simulink model "Sim_Control_Dezvoltare"  (R2022b)
settings: Solver=VariableStepAuto  StartTime=0.0  StopTime=400  RelTol=1e-3
values from neighbouring files (symbols this model uses):
  g = 9.80665    [Date_initializare_SIM.m]
  h = 0.30    (= 0.3)    [Date_initializare_SIM.m]
undefined symbols (not defined in the file or in its folder): X, Y, Z
libraries: sm_lib x175, nesl_utility x70, slpidlib x2
(part 1 of 5)
settings Model: PacingRate=1.100000  Creator=MUN  LastModifiedBy=MUN

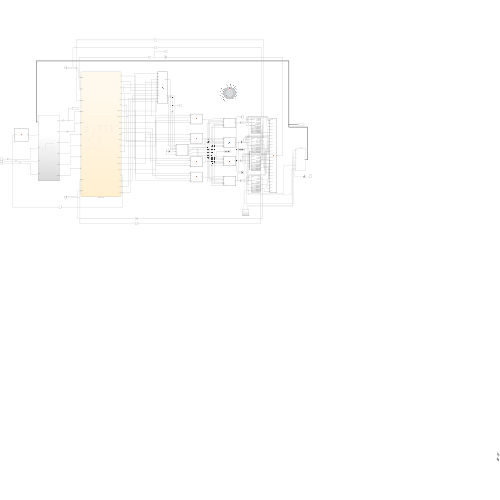
[thumbnail: Simulink's stored preview of the top-level diagram]
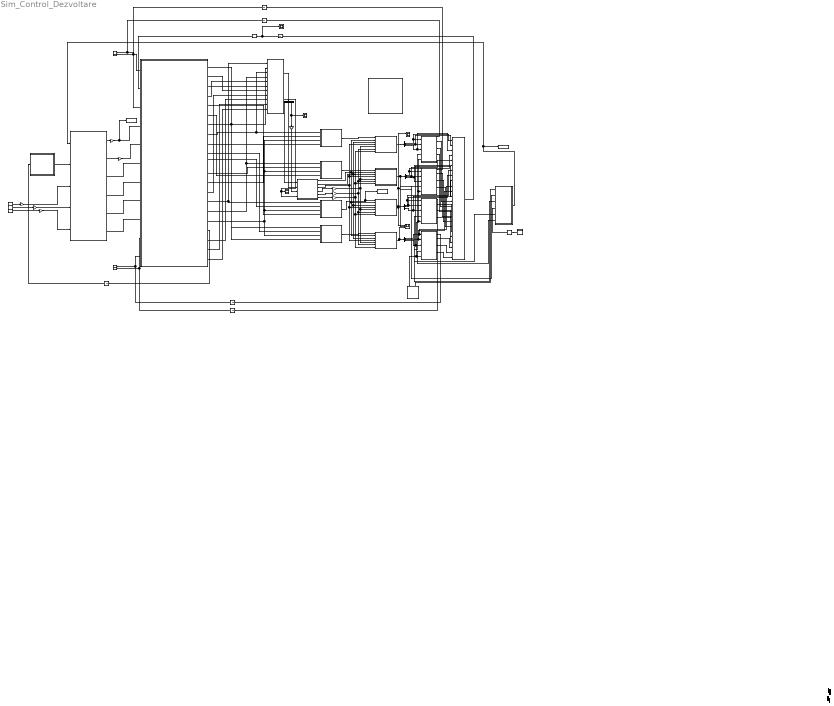
== system Sim_Control_Dezvoltare ==
  Abs2 : Abs  SaturateOnIntegerOverflow=off
  Constant12 : Constant  Value=-0.966540570841012  SampleTime=0.01
  Constant13 : Constant  Value=0.001  SampleTime=0.01
  Constant14 : Constant  Value=0.001  SampleTime=0.01
  Demux{10..14} (5 alike) : Demux  Outputs=3
  Gain{,1..4} (5 alike) : Gain
  Gain{5..8} (4 alike) : Gain  Gain=0
  Knob6 : KnobBlock  ScaleMin=-40  ScaleMax=40
  MATLAB Function1 : MATLAB Function  TreatAsAtomicUnit=on
  MATLAB Function18 : MATLAB Function  TreatAsAtomicUnit=on
  MATLAB Function22 : MATLAB Function  TreatAsAtomicUnit=on
  MATLAB Function23 : MATLAB Function  TreatAsAtomicUnit=on
  MATLAB Function24 : MATLAB Function  TreatAsAtomicUnit=on
  MATLAB Function25 : MATLAB Function  TreatAsAtomicUnit=on
  MATLAB Function26 : MATLAB Function  TreatAsAtomicUnit=on
  MATLAB Function28 : MATLAB Function  TreatAsAtomicUnit=on
  MATLAB Function29 : MATLAB Function  TreatAsAtomicUnit=on
  MATLAB Function5 : MATLAB Function  TreatAsAtomicUnit=on
  MATLAB Function6 : MATLAB Function  TreatAsAtomicUnit=on
  MATLAB Function7 : MATLAB Function  TreatAsAtomicUnit=on
  Mux{2..7} (6 alike) : Mux  Inputs=2
  Scope1 : Scope
  Scope2 : Scope  NumInputPorts=2
  Scope3 : Scope  NumInputPorts=2
  Scope4 : Scope
  Scope5 : Scope  NumInputPorts=2
  Scope8 : Scope
  Scope9 : Scope  NumInputPorts=3
  Step Planning Logic3 : Stateflow chart  TreatAsAtomicUnit=on
      settings: PortSchema="{\"entries\":[{\"content\":{\"sides\":[{\"content\":{\"connectorIds\":[\"In6\",\"In7\",\"In5\",\"In1\",\"In2\",\"In8\",\"In9\",\"In10\",\"In11\",\"In3\",\"In4\"]},\"type\":\"ConnectorPlacement.EquallySpacedRectSide\",\"uuid\":\"67f320ed-e42e-4d7a-9e62-e653fd80f8e7\"},{\"content\":{\"connectorIds\":[\"Out8\",\"Out9\",\"Out10\",\"Out11\",\"Out5\",\"Out6\",\"Out14\",\"Out15\",\"Out3\",\"Out2\",\"Out1\",\"Out4\",\"Out7\",\"Out12\",\"Out13\",\"Out16\",\"Out17\",\"Out18\",\"Out19\",\"Out20\",\"Out21\"],\"side\":\"RIGHT\"},\"type\":\"ConnectorPlacement.EquallySpacedRectSide\",\"uuid\":\"e3cd9553-5eec-4090-9ce7-ca96f0786c72\"},{\"content\":{\"connectorIds\":[],\"side\":\"TOP\"},\"type\":\"ConnectorPlacement.EquallySpacedRectSide\",\"uuid\":\"81deb129-37ff-4d08-a927-1694f21adb89\"}]},\"type\":\"ConnectorPlacement.EquallySpacedConnector\",\"uuid\":\"ac0f76e8-4d76-423d-ab5b-73feabaa903f\"}],\"packageUris\":[\"http://schema.mathworks.com/mf0/Connector/R2020b\"],\"version\":\"1.0\"}"
  Subsystem13 : Subsystem
  Subsystem14 : Subsystem
  Subsystem16 : Subsystem
  Subsystem17 : Subsystem
  Subsystem18 : Subsystem
  Subsystem19 : Subsystem
  To Workspace1 : ToWorkspace  VariableName=simout  SaveFormat=Timeseries  SampleTime=-1
  To Workspace2 : ToWorkspace  VariableName=simout1  SaveFormat=Timeseries  SampleTime=-1
  To Workspace3 : ToWorkspace  VariableName=simout2  SampleTime=1
  To Workspace4 : ToWorkspace  VariableName=simout3  SampleTime=1
  Unit Delay{8..13} (6 alike) : UnitDelay  SampleTime=-1  HasFrameUpgradeWarning=on
  imu_joint3 : sm_lib/Joints/Weld Joint  JointMode=Normal  SenseConstraintForce=off  SenseConstraintForceX=off  SenseConstraintForceY=off  SenseConstraintForceZ=off  SenseConstraintTorque=off  SenseConstraintTorqueX=off  SenseConstraintTorqueY=off  SenseConstraintTorqueZ=off  SenseTotalForce=off  SenseTotalForceX=off  SenseTotalForceY=off  SenseTotalForceZ=off  SenseTotalTorque=off  SenseTotalTorqueX=off  SenseTotalTorqueY=off  SenseTotalTorqueZ=off  CompositeWrenchDir=FollowerOnBase  CompositeWrenchFrame=BaseFrame
  imu_link3 : Subsystem
  trunk3 : Subsystem
      settings: PortSchema="{\"entries\":[{\"content\":{\"sides\":[{\"content\":{\"connectorIds\":[\"Out1\"]},\"type\":\"ConnectorPlacement.EquallySpacedRectSide\",\"uuid\":\"7376a86a-8770-43a1-89a9-4e7813322353\"},{\"content\":{\"connectorIds\":[\"RConn1\",\"RConn2\",\"RConn3\",\"RConn4\",\"RConn5\",\"RConn6\"],\"side\":\"RIGHT\"},\"type\":\"ConnectorPlacement.EquallySpacedRectSide\",\"uuid\":\"180eba54-5c89-4d6d-8e58-15143fb194fc\"},{\"content\":{\"connectorIds\":[],\"side\":\"TOP\"},\"type\":\"ConnectorPlacement.EquallySpacedRectSide\",\"uuid\":\"86808b5f-7587-4320-85a4-2335862b1c59\"}]},\"type\":\"ConnectorPlacement.EquallySpacedConnector\",\"uuid\":\"b1910719-1a28-43ea-8867-88a05065806a\"}],\"packageUris\":[\"http://schema.mathworks.com/mf0/Connector/R2020b\"],\"version\":\"1.0\"}"
  wires:
  MATLAB Function26/6(Rz) -> Gain4/1
  MATLAB Function6/1(q_hl) -> Scope9/3, Demux13/1
  MATLAB Function26/5(Ry) -> Gain1/1
  Subsystem18/1(Fn_RR) -> Unit Delay10/1
  Step Planning Logic3/13(footRH_prev) -> MATLAB Function18/1(Fr), MATLAB Function28/1(A)
  Step Planning Logic3/18(step) -> Unit Delay12/1
  Step Planning Logic3/6(dLB) -> MATLAB Function23/4(d)
  MATLAB Function28/1(X) -> To Workspace4/1, MATLAB Function1/1(pstar)
  Step Planning Logic3/12(pfl) -> MATLAB Function18/8(pfl)
  Step Planning Logic3/10(prl) -> MATLAB Function18/6(prl)
  MATLAB Function26/4(Rx) -> Gain/1
  Constant13/1 -> Gain7/1
  Demux14/3 -> Subsystem19/3(Q_CALF_RL), MATLAB Function29/6(Ce_C_RL)
  Constant14/1 -> Gain6/1
  Subsystem19/3(QS_HIP_RL) -> MATLAB Function29/16(Se_H_RL)
  MATLAB Function5/1(q_br) -> Demux12/1
  Constant12/1 -> Gain8/1
  Subsystem14/6(QS_THIGH_FR) -> MATLAB Function29/20(Se_T_FR)
  Subsystem16/6(QS_THIGH_FL) -> MATLAB Function29/23(Se_T_FL)
  Demux11/2 -> MATLAB Function29/8(Ce_T_FR), Subsystem14/2(Q_THIGH_FR)
  Demux12/1 -> Subsystem18/1(Q_HIP_RR), MATLAB Function29/1(Ce_H_RR)
  Subsystem19/9(QS_CALF_RL) -> MATLAB Function29/18(Se_C_RL)
  MATLAB Function29/1(E) -> Unit Delay13/1
  Unit Delay13/1 -> Scope8/1, Abs2/1
  Gain2/1 -> Step Planning Logic3/2(stepLat)
  Abs2/1 -> Step Planning Logic3/7(err_cg)
  Gain3/1 -> To Workspace1/1, Step Planning Logic3/1(stepFwd)
  Step Planning Logic3/2(footLH) -> MATLAB Function22/2(B)
  Demux11/3 -> MATLAB Function29/9(Ce_C_FR), Subsystem14/3(Q_CALF_FR)
  Subsystem16/9(QS_CALF_FL) -> MATLAB Function29/24(Se_C_FL)
  Subsystem18/9(QS_CALF_RR) -> MATLAB Function29/15(Se_C_RR)
  Subsystem19/6(QS_THIGH_RL) -> MATLAB Function29/17(Se_T_RL)
  Unit Delay11/1 -> Step Planning Logic3/6(presRL), Scope3/2
  Subsystem14/9(QS_CALF_FR) -> MATLAB Function29/21(Se_C_FR)
  Unit Delay9/1 -> Scope2/2, Step Planning Logic3/3(presFR)
  MATLAB Function24/1(X) -> MATLAB Function5/1(pstar)
  Subsystem14/3(QS_HIP_FR) -> MATLAB Function29/19(Se_H_FR)
  Demux12/3 -> MATLAB Function29/3(Ce_C_RR), Subsystem18/3(Q_CALF_RR)
  Subsystem18/3(QS_HIP_RR) -> MATLAB Function29/13(Se_H_RR)
  Subsystem16/3(QS_HIP_FL) -> MATLAB Function29/22(Se_H_FL)
  Step Planning Logic3/5(dRH) -> MATLAB Function28/4(d)
  Unit Delay10/1 -> Scope3/1, Step Planning Logic3/5(presRR)
  Demux13/3 -> Subsystem16/3(Q_CALF_FL), MATLAB Function29/12(Ce_C_FL)
  Subsystem13/2(posOut1) -> Gain2/1
  Demux14/1 -> MATLAB Function29/4(Ce_H_RL), Subsystem19/1(Q_HIP_RL)
  MATLAB Function18/1(centroid) -> Demux10/1
  MATLAB Function22/1(X1) -> MATLAB Function6/1(pstar)
  Step Planning Logic3/9(prr) -> MATLAB Function18/7(prr)
  Subsystem13/1(posOut) -> Gain3/1
  Subsystem14/1(Fn_FR) -> Unit Delay9/1
  Step Planning Logic3/4(footLB) -> MATLAB Function23/2(B)
  Demux13/2 -> MATLAB Function29/11(Ce_T_FL), Subsystem16/2(Q_THIGH_FL)
  Demux10/1 -> MATLAB Function26/1(X)
  Demux14/2 -> MATLAB Function29/5(Ce_T_RL), Subsystem19/2(Q_THIGH_RL)
  Step Planning Logic3/7(dRB) -> MATLAB Function24/4(d)
  Unit Delay8/1 -> Scope2/1, Step Planning Logic3/4(presFL)
  Demux12/2 -> Subsystem18/2(Q_THIGH_RR), MATLAB Function29/2(Ce_T_RR)
  Subsystem19/1(Fn_RL) -> Unit Delay11/1
  Step Planning Logic3/16(footLB_prev) -> MATLAB Function18/4(Rl), MATLAB Function23/1(A)
  Demux10/2 -> MATLAB Function26/2(Y)
  Demux13/1 -> MATLAB Function29/10(Ce_H_FL), Subsystem16/1(Q_HIP_FL)
  Subsystem16/1(Fn_FL) -> Unit Delay8/1
  Unit Delay12/1 -> MATLAB Function25/1(step)
  Step Planning Logic3/1(footRH) -> MATLAB Function28/2(B)
  Step Planning Logic3/15(footRB_prev) -> MATLAB Function18/3(Rr), MATLAB Function24/1(A)
  MATLAB Function23/1(X) -> MATLAB Function7/1(pstar)
  Step Planning Logic3/8(dLH) -> MATLAB Function22/4(d)
  trunk3/1(meas) -> Subsystem13/1(In1), To Workspace2/1
  Step Planning Logic3/14(footLH_prev) -> MATLAB Function18/2(Fl), MATLAB Function22/1(A)
  Subsystem18/6(QS_THIGH_RR) -> MATLAB Function29/14(Se_T_RR)
  Step Planning Logic3/11(pfr) -> MATLAB Function18/5(pfr)
  Step Planning Logic3/3(footRB) -> MATLAB Function24/2(B)
  MATLAB Function25/1(traj) -> Subsystem13/2(traj)
  MATLAB Function7/1(q_bl) -> Demux14/1, Scope9/2
  Step Planning Logic3/19(rx_out) -> MATLAB Function18/9(rx)
  Step Planning Logic3/20(ry_out) -> MATLAB Function18/10(ry)
  Step Planning Logic3/21(rz_out) -> MATLAB Function18/11(rz)
  Gain/1 -> MATLAB Function5/5(Rx), MATLAB Function7/5(Rx), MATLAB Function6/5(Rx), MATLAB Function1/5(Rx)
  Gain1/1 -> MATLAB Function5/6(Ry), MATLAB Function7/6(Ry), MATLAB Function6/6(Ry), MATLAB Function1/6(Ry)
  Gain4/1 -> MATLAB Function5/7(Rz), MATLAB Function7/7(Rz), MATLAB Function1/7(Rz), MATLAB Function6/7(Rz)
  Subsystem13/3(posOut2) -> Step Planning Logic3/8(R)
  Step Planning Logic3/17(timp_traj) -> MATLAB Function24/3(t), MATLAB Function23/3(t), MATLAB Function28/3(t), MATLAB Function22/3(t)
  Demux10/3 -> Gain5/1, Scope1/1
  Gain5/1 -> MATLAB Function26/3(Z)
  Gain6/1 -> Subsystem13/3(R_com)
  Gain7/1 -> Subsystem13/4(R_com1)
  Gain8/1 -> Subsystem13/5(R_com2)
  Subsystem13/6(posOut5) -> Step Planning Logic3/11(rz)
  Subsystem13/5(posOut4) -> Step Planning Logic3/10(ry)
  Subsystem13/4(posOut3) -> Step Planning Logic3/9(rx)
  MATLAB Function18/2(rot) -> Scope4/1, MATLAB Function26/4(R)
  MATLAB Function1/1(q_r) -> Scope5/1, To Workspace3/1, Demux11/1, Scope9/1
  MATLAB Function26/1(Tx) -> MATLAB Function5/2(Tx), MATLAB Function6/2(Tx), MATLAB Function1/2(Tx), MATLAB Function7/2(Tx)
  MATLAB Function26/2(Ty) -> MATLAB Function5/3(Ty), MATLAB Function6/3(Ty), MATLAB Function1/3(Ty), MATLAB Function7/3(Ty)
  MATLAB Function26/3(Tz) -> MATLAB Function5/4(Tz), MATLAB Function7/4(Tz), MATLAB Function6/4(Tz), MATLAB Function1/4(Tz)
  Demux11/1 -> MATLAB Function29/7(Ce_H_FR), Subsystem14/1(Q_HIP_FR)
  connections:
  Subsystem17/LConn1 -- Subsystem19/LConn2 -- Subsystem18/LConn2 -- Subsystem14/LConn2 -- Subsystem16/LConn2
  Subsystem17/LConn2 -- trunk3/RConn6
  Subsystem14/LConn1 -- trunk3/RConn2
  Subsystem16/LConn1 -- trunk3/RConn1
  imu_joint3/LConn1 -- trunk3/RConn3
  imu_joint3/RConn1 -- imu_link3/LConn1
  Subsystem19/LConn1 -- trunk3/RConn5
  Subsystem18/LConn1 -- trunk3/RConn4

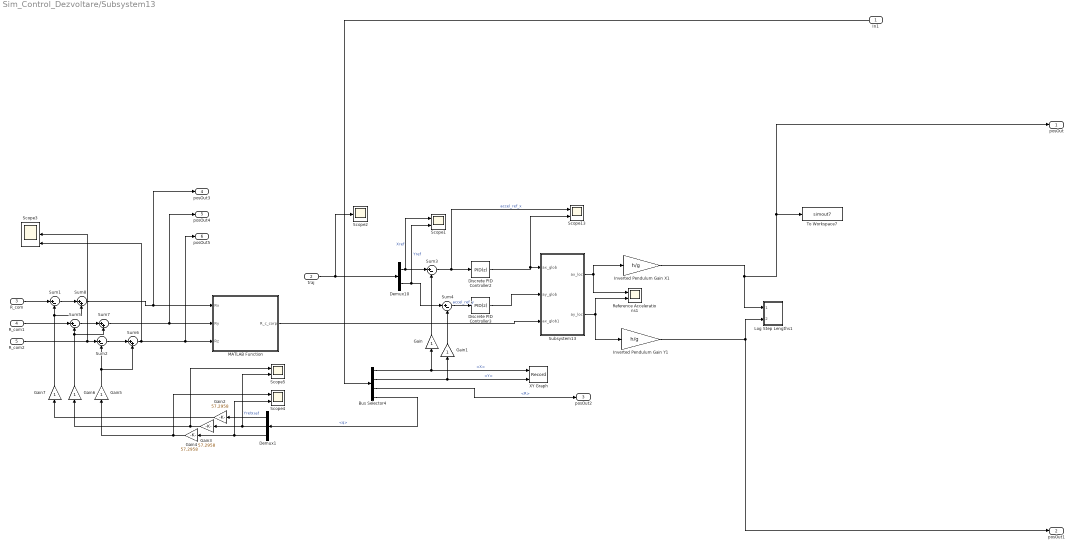
== system Sim_Control_Dezvoltare/Subsystem13 ==
  In1 : Inport
  traj : Inport  Port=2
  R_com : Inport  Port=3
  R_com1 : Inport  Port=4
  R_com2 : Inport  Port=5
  Bus Selector4 : BusSelector  OutputSignals=X,Y,R,q
  Demux1 : Demux  Outputs=3
  Demux10 : Demux  Outputs=2
  Discrete PID Controller2 : slpidlib/PID Controller  Controller=PID  Form=Parallel  TimeDomain=Discrete-time  UseExternalTs=off  SampleTime=-1  IntegratorMethod=Forward Euler  FilterMethod=Forward Euler  ControllerParametersSource=internal  P=1  I=0  UseKiTs=off  D=0  N=100  UseFilter=off  TunerSelectOption=Transfer Function Based (PID Tuner App)  InitialConditionSource=internal  InitialConditionForIntegrator=0  InitialConditionForFilter=0  DifferentiatorICPrevScaledInput=0  ExternalReset=none  TrackingMode=off  Kt=1  LimitOutput=off  SatLimitsSource=internal  UpperSaturationLimit=inf  LowerSaturationLimit=-inf  LinearizeAsGain=off  AntiWindupMode=none  Kb=1  LimitIntegrator=off  UpperIntegratorSaturationLimit=inf  LowerIntegratorSaturationLimit=-inf  POutMin=[]  POutMax=[]  IOutMin=[]  IOutMax=[]  DOutMin=[]  DOutMax=[]  NOutMin=[]  NOutMax=[]  SumOutMin=[]  SumOutMax=[]  SaturationOutMin=[]  SaturationOutMax=[]  PParamMin=[]  PParamMax=[]  IParamMin=[]  IParamMax=[]  DParamMin=[]  DParamMax=[]  NParamMin=[]  NParamMax=[]  KbParamMin=[]  KbParamMax=[]  KtParamMin=[]  KtParamMax=[]  KbOutMin=[]  KbOutMax=[]  KtOutMin=[]  KtOutMax=[]  IntegratorOutMin=[]  IntegratorOutMax=[]  FilterOutMin=[]  FilterOutMax=[]  SumI1OutMin=[]  SumI1OutMax=[]  SumI2OutMin=[]  SumI2OutMax=[]  SumI3OutMin=[]  SumI3OutMax=[]  SumI4OutMin=[]  SumI4OutMax=[]  SumDOutMin=[]  SumDOutMax=[]  DifferentiatorOutMin=[]  DifferentiatorOutMax=[]  FilterDiffOutCoefMin=[]  FilterDiffOutCoefMax=[]  ReciprocalOutMin=[]  ReciprocalOutMax=[]  SumDenOutMin=[]  SumDenOutMax=[]  SumNumOutMin=[]  SumNumOutMax=[]  DivideOutMin=[]  DivideOutMax=[]  UdiffTsProdOutMin=[]  UdiffTsProdOutMax=[]  NTsProdOutMin=[]  NTsProdOutMax=[]  UintegralTsProdOutMin=[]  UintegralTsProdOutMax=[]  UngainTsProdOutMin=[]  UngainTsProdOutMax=[]  ClampingZeroOutDataTypeStr=Inherit: Inherit via back propagation  ClampingZeroOutMin=[]  ClampingZeroOutMax=[]  FilterDenConstantOutDataTypeStr=Inherit: Inherit via back propagation  FilterDenConstantOutMin=[]  FilterDenConstantOutMax=[]  PCopyOutDataTypeStr=Inherit: Inherit via back propagation  PCopyOutMin=[]  PCopyOutMax=[]  NCopyOutDataTypeStr=Inherit: Inherit via back propagation  NCopyOutMin=[]  NCopyOutMax=[]  IntegratorContinuousStateAttributes=''  IntegratorStateMustResolveToSignalObject=off  IntegratorRTWStateStorageClass=Auto  FilterContinuousStateAttributes=''  FilterStateMustResolveToSignalObject=off  FilterRTWStateStorageClass=Auto  ParallelPVariant=InternalParameters  IdealPVariant=Disabled  IVariant=InternalParameters  DVariant=InternalParameters  IntegratorVariant=Discrete  SatVariant=Disabled  AWVariant=Passthrough  PCopyVariant=Disabled  TRVariant=Disabled  FdbkBlocksVariant=Forward  IdealPFdbkVariant=Disabled  SatFdbkVariant=Disabled  DerivativeFilterVariant=Differentiator  NVariant=Passthrough  NCopyVariant=Disabled_SignalSpec  FilterICVariant=InternalICsDifferentiator  IntegratorICVariant=InternalICs  ExternalResetVariant=Disabled  TRSumVariant=Passthrough  SumFdbkVariant=Disabled  SumVariant=Sum_PID  TsampFilterVariant=InternalTs  TsampNgainVariant=Passthrough  TsampIntegralVariant=Passthrough  ExternalSaturationOutDataTypeStr=Inherit: Same as second input
      settings: LibrarySourceBlock=simulink/Discrete/Discrete PID Controller
  Discrete PID Controller3 : slpidlib/PID Controller  Controller=PID  Form=Parallel  TimeDomain=Discrete-time  UseExternalTs=off  SampleTime=-1  IntegratorMethod=Forward Euler  FilterMethod=Forward Euler  ControllerParametersSource=internal  P=1  I=0  UseKiTs=off  D=0  N=100  UseFilter=off  TunerSelectOption=Transfer Function Based (PID Tuner App)  InitialConditionSource=internal  InitialConditionForIntegrator=0  InitialConditionForFilter=0  DifferentiatorICPrevScaledInput=0  ExternalReset=none  TrackingMode=off  Kt=1  LimitOutput=off  SatLimitsSource=internal  UpperSaturationLimit=inf  LowerSaturationLimit=-inf  LinearizeAsGain=off  AntiWindupMode=none  Kb=1  LimitIntegrator=off  UpperIntegratorSaturationLimit=inf  LowerIntegratorSaturationLimit=-inf  POutMin=[]  POutMax=[]  IOutMin=[]  IOutMax=[]  DOutMin=[]  DOutMax=[]  NOutMin=[]  NOutMax=[]  SumOutMin=[]  SumOutMax=[]  SaturationOutMin=[]  SaturationOutMax=[]  PParamMin=[]  PParamMax=[]  IParamMin=[]  IParamMax=[]  DParamMin=[]  DParamMax=[]  NParamMin=[]  NParamMax=[]  KbParamMin=[]  KbParamMax=[]  KtParamMin=[]  KtParamMax=[]  KbOutMin=[]  KbOutMax=[]  KtOutMin=[]  KtOutMax=[]  IntegratorOutMin=[]  IntegratorOutMax=[]  FilterOutMin=[]  FilterOutMax=[]  SumI1OutMin=[]  SumI1OutMax=[]  SumI2OutMin=[]  SumI2OutMax=[]  SumI3OutMin=[]  SumI3OutMax=[]  SumI4OutMin=[]  SumI4OutMax=[]  SumDOutMin=[]  SumDOutMax=[]  DifferentiatorOutMin=[]  DifferentiatorOutMax=[]  FilterDiffOutCoefMin=[]  FilterDiffOutCoefMax=[]  ReciprocalOutMin=[]  ReciprocalOutMax=[]  SumDenOutMin=[]  SumDenOutMax=[]  SumNumOutMin=[]  SumNumOutMax=[]  DivideOutMin=[]  DivideOutMax=[]  UdiffTsProdOutMin=[]  UdiffTsProdOutMax=[]  NTsProdOutMin=[]  NTsProdOutMax=[]  UintegralTsProdOutMin=[]  UintegralTsProdOutMax=[]  UngainTsProdOutMin=[]  UngainTsProdOutMax=[]  ClampingZeroOutDataTypeStr=Inherit: Inherit via back propagation  ClampingZeroOutMin=[]  ClampingZeroOutMax=[]  FilterDenConstantOutDataTypeStr=Inherit: Inherit via back propagation  FilterDenConstantOutMin=[]  FilterDenConstantOutMax=[]  PCopyOutDataTypeStr=Inherit: Inherit via back propagation  PCopyOutMin=[]  PCopyOutMax=[]  NCopyOutDataTypeStr=Inherit: Inherit via back propagation  NCopyOutMin=[]  NCopyOutMax=[]  IntegratorContinuousStateAttributes=''  IntegratorStateMustResolveToSignalObject=off  IntegratorRTWStateStorageClass=Auto  FilterContinuousStateAttributes=''  FilterStateMustResolveToSignalObject=off  FilterRTWStateStorageClass=Auto  ParallelPVariant=InternalParameters  IdealPVariant=Disabled  IVariant=InternalParameters  DVariant=InternalParameters  IntegratorVariant=Discrete  SatVariant=Disabled  AWVariant=Passthrough  PCopyVariant=Disabled  TRVariant=Disabled  FdbkBlocksVariant=Forward  IdealPFdbkVariant=Disabled  SatFdbkVariant=Disabled  DerivativeFilterVariant=Differentiator  NVariant=Passthrough  NCopyVariant=Disabled_SignalSpec  FilterICVariant=InternalICsDifferentiator  IntegratorICVariant=InternalICs  ExternalResetVariant=Disabled  TRSumVariant=Passthrough  SumFdbkVariant=Disabled  SumVariant=Sum_PID  TsampFilterVariant=InternalTs  TsampNgainVariant=Passthrough  TsampIntegralVariant=Passthrough  ExternalSaturationOutDataTypeStr=Inherit: Same as second input
      settings: LibrarySourceBlock=simulink/Discrete/Discrete PID Controller
  Gain{,1,5..7} (5 alike) : Gain
  Gain2 : Gain  Gain=57.2958
  Gain3 : Gain  Gain=57.2958
  Gain4 : Gain  Gain=57.2958
  Inverted Pendulum Gain X1 : Gain  Gain=h/g
  Inverted Pendulum Gain Y1 : Gain  Gain=h/g
  Log Step Lengths1 : Subsystem
  MATLAB Function : MATLAB Function  TreatAsAtomicUnit=on
  Reference Accelerations1 : Scope  NumInputPorts=2
  Scope{1,4..5,13} (4 alike) : Scope  NumInputPorts=2
  Scope2 : Scope
  Scope3 : Scope  NumInputPorts=3
  Subsystem13 : Subsystem
  Sum{1..5} (5 alike) : Sum  Inputs=|+-
  Sum6 : Sum  Inputs=|++
  Sum7 : Sum  Inputs=|++
  Sum8 : Sum  Inputs=|++
  To Workspace7 : ToWorkspace  VariableName=simout7  SaveFormat=Timeseries  SampleTime=-1
  XY Graph : Record  FileSettingsInternal="{\"entries\":[{\"content\":{\"excelSettings\":{\"content\":{},\"type\":\"Streamout.ExcelSettings\"}},\"type\":\"Streamout.FileSettingStorage\",\"uuid\":\"21eb5009-1c1e-4216-b0f2-44376c94cc54\"}],\"packageUris\":[\"http://schema.mathworks.com/mf0/streamout_blocks/R2020a\"],\"version\":\"1.0\"}"  Layout=[1 1]  SignalsInternal="{\"entries\":[{\"content\":{\"signals\":[{\"content\":{\"blockPath\":[\"Sim_Control_Dezvoltare/Subsystem13/XY Graph\"],\"channel\":[],\"dimensions\":[1],\"domain\":\"Sim_Control_Dezvoltare/Subsystem13/XY Graph\",\"lineColor\":\"#4dbeee\",\"plots\":[],\"port\":1,\"sid\":[\"\"],\"signalID\":77,\"signalName\":\"<X>\"},\"type\":\"RecordBlkView.Signal\",\"uuid\":\"adf75aa9-499f-41cd-acc2-b4045e37f077\"},{\"content\":{\"blockPath\":[\"Sim_Control_Dezvoltare/Subsystem13/XY Graph\"],\"channel\":[],\"dimensions\":[1],\"domain\":\"Sim_Control_Dezvoltare/Subsystem13/XY Graph\",\"lineColor\":\"#a2142f\",\"plots\":[],\"port\":2,\"sid\":[\"\"],\"signalID\":81,\"signalName\":\"<Y>\"},\"type\":\"RecordBlkView.Signal\",\"uuid\":\"65bc2fbe-db19-4d53-b60a-250f9e7712ce\"}]},\"type\":\"RecordBlkView.InputSignals\",\"uuid\":\"d318ff41-ac82-4101-83f6-c3a9333ec2b0\"}],\"packageUris\":[\"http://schema.mathworks.com/mf0/streamout_blocks/R2020a\"],\"version\":\"1.0\"}"  VisualizationBindings="{\"xyplotplugin\":{\"info\":[{\"series\":[],\"subplotID\":1}]}}"  CompatibilityTag=XY
  posOut : Outport
  posOut1 : Outport  Port=2
  posOut2 : Outport  Port=3
  posOut3 : Outport  Port=4
  posOut4 : Outport  Port=5
  posOut5 : Outport  Port=6
  wires:
  Demux10/1 -> Scope1/1, Sum3/1  "Xref"
  Demux10/2 -> Scope1/2, Sum4/1  "Yref"
  Bus Selector4/2 -> XY Graph/2, Gain1/1  "<Y>"
  Subsystem13/2(ay_loc) -> Inverted Pendulum Gain Y1/1, Reference Accelerations1/2
  Sum4/1 -> Discrete PID Controller3/1  "accel_ref_y"
  Subsystem13/1(ax_loc) -> Reference Accelerations1/1, Inverted Pendulum Gain X1/1
  Bus Selector4/1 -> XY Graph/1, Gain/1  "<X>"
  In1/1 -> Bus Selector4/1
  Sum3/1 -> Discrete PID Controller2/1, Scope13/1  "accel_ref_x"
  Inverted Pendulum Gain X1/1 -> Log Step Lengths1/1(stepFwd), posOut/1, To Workspace7/1
  Discrete PID Controller3/1 -> Subsystem13/2(ay_glob)
  Discrete PID Controller2/1 -> Subsystem13/1(ax_glob), Scope13/2
  Inverted Pendulum Gain Y1/1 -> posOut1/1, Log Step Lengths1/2(stepLat)
  traj/1 -> Scope2/1, Demux10/1
  Gain/1 -> Sum3/2
  Gain1/1 -> Sum4/2
  Bus Selector4/4 -> Demux1/1  "<q>"
  R_com/1 -> Sum1/1
  R_com1/1 -> Sum5/1
  R_com2/1 -> Scope3/2, Sum2/1
  MATLAB Function/1(R_c_corp) -> Subsystem13/3(ax_glob1)
  Demux1/2 -> Scope5/2, Gain3/1  "Yref"
  Demux1/1 -> Gain2/1  "Xref"
  Demux1/3 -> Gain4/1, Scope4/2
  Gain2/1 -> Gain7/1
  Gain3/1 -> Gain6/1, Scope5/1
  Bus Selector4/3 -> posOut2/1  "<R>"
  Gain5/1 -> Sum6/2, Sum2/2
  Gain6/1 -> Sum5/2, Sum7/2
  Gain7/1 -> Sum8/2, Sum1/2
  Sum6/1 -> posOut5/1, MATLAB Function/3(Rz), Scope3/3
  Sum2/1 -> Sum6/1
  Gain4/1 -> Scope4/1, Gain5/1
  Sum5/1 -> Sum7/1
  Sum7/1 -> posOut4/1, MATLAB Function/2(Ry)
  Sum1/1 -> Sum8/1
  Sum8/1 -> posOut3/1, MATLAB Function/1(Rx)

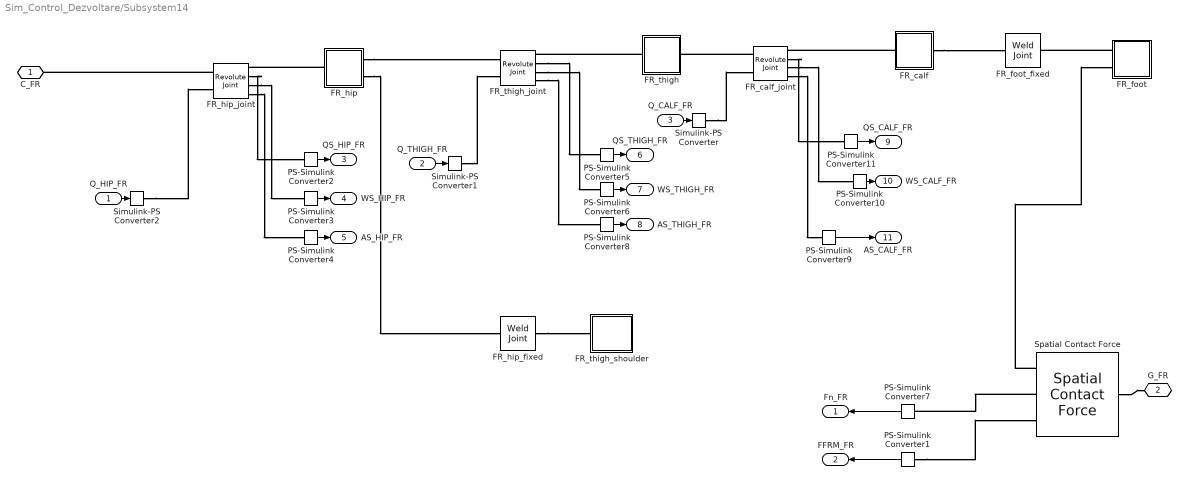
== system Sim_Control_Dezvoltare/Subsystem14 ==
  Q_HIP_FR : Inport
  Q_THIGH_FR : Inport  Port=2
  Q_CALF_FR : Inport  Port=3
  FR_calf : Subsystem
  FR_calf_joint : sm_lib/Joints/Revolute Joint  JointMode=Normal  SenseConstraintForce=off  SenseConstraintForceX=off  SenseConstraintForceY=off  SenseConstraintForceZ=off  SenseConstraintTorque=off  SenseConstraintTorqueX=off  SenseConstraintTorqueY=off  SenseConstraintTorqueZ=off  SenseTotalForce=off  SenseTotalForceX=off  SenseTotalForceY=off  SenseTotalForceZ=off  SenseTotalTorque=off  SenseTotalTorqueX=off  SenseTotalTorqueY=off  SenseTotalTorqueZ=off  CompositeWrenchDir=FollowerOnBase  CompositeWrenchFrame=BaseFrame  EquilibriumPosition=0  EquilibriumPositionUnits=deg  SpringStiffness=0  SpringStiffnessUnits=N*m/deg  DampingCoefficient=0.01  DampingCoefficientUnits=kg*m^2/(rad*s)  TorqueActuationMode=ComputedTorque  MotionActuationMode=InputMotion  SensePosition=on  SenseVelocity=on  SenseAcceleration=on  SenseTorqueForce=off  SenseLowerLimitTorqueForce=off  SenseUpperLimitTorqueForce=off  LowerLimitSpecify=on  LowerLimitBound=-2.69653369433  LowerLimitBoundUnits=rad  LowerLimitStiffness=1e4  LowerLimitStiffnessUnits=N*m/deg  LowerLimitDamping=10  LowerLimitDampingUnits=N*m/(deg/s)  LowerLimitTransitionRegionWidth=0.1  LowerLimitTransitionRegionWidthUnits=deg  UpperLimitSpecify=on  UpperLimitBound=-0.916297857297  UpperLimitBoundUnits=rad  UpperLimitStiffness=1e4  UpperLimitStiffnessUnits=N*m/deg  UpperLimitDamping=10  UpperLimitDampingUnits=N*m/(deg/s)  UpperLimitTransitionRegionWidth=0.1  UpperLimitTransitionRegionWidthUnits=deg  PositionTargetSpecify=on  PositionTargetPriority=High  PositionTargetValue=-1.7298  PositionTargetValueUnits=rad  VelocityTargetSpecify=off  VelocityTargetPriority=High  VelocityTargetValue=1  VelocityTargetValueUnits=deg/s
  FR_foot : Subsystem
  FR_foot_fixed : sm_lib/Joints/Weld Joint  JointMode=Normal  SenseConstraintForce=off  SenseConstraintForceX=off  SenseConstraintForceY=off  SenseConstraintForceZ=off  SenseConstraintTorque=off  SenseConstraintTorqueX=off  SenseConstraintTorqueY=off  SenseConstraintTorqueZ=off  SenseTotalForce=off  SenseTotalForceX=off  SenseTotalForceY=off  SenseTotalForceZ=off  SenseTotalTorque=off  SenseTotalTorqueX=off  SenseTotalTorqueY=off  SenseTotalTorqueZ=off  CompositeWrenchDir=FollowerOnBase  CompositeWrenchFrame=BaseFrame
  FR_hip : Subsystem
  FR_hip_fixed : sm_lib/Joints/Weld Joint  JointMode=Normal  SenseConstraintForce=off  SenseConstraintForceX=off  SenseConstraintForceY=off  SenseConstraintForceZ=off  SenseConstraintTorque=off  SenseConstraintTorqueX=off  SenseConstraintTorqueY=off  SenseConstraintTorqueZ=off  SenseTotalForce=off  SenseTotalForceX=off  SenseTotalForceY=off  SenseTotalForceZ=off  SenseTotalTorque=off  SenseTotalTorqueX=off  SenseTotalTorqueY=off  SenseTotalTorqueZ=off  CompositeWrenchDir=FollowerOnBase  CompositeWrenchFrame=BaseFrame
  FR_hip_joint : sm_lib/Joints/Revolute Joint  JointMode=Normal  SenseConstraintForce=off  SenseConstraintForceX=off  SenseConstraintForceY=off  SenseConstraintForceZ=off  SenseConstraintTorque=off  SenseConstraintTorqueX=off  SenseConstraintTorqueY=off  SenseConstraintTorqueZ=off  SenseTotalForce=off  SenseTotalForceX=off  SenseTotalForceY=off  SenseTotalForceZ=off  SenseTotalTorque=off  SenseTotalTorqueX=off  SenseTotalTorqueY=off  SenseTotalTorqueZ=off  CompositeWrenchDir=FollowerOnBase  CompositeWrenchFrame=BaseFrame  EquilibriumPosition=0  EquilibriumPositionUnits=deg  SpringStiffness=0  SpringStiffnessUnits=N*m/deg  DampingCoefficient=0.01  DampingCoefficientUnits=kg*m^2/(rad*s)  TorqueActuationMode=ComputedTorque  MotionActuationMode=InputMotion  SensePosition=on  SenseVelocity=on  SenseAcceleration=on  SenseTorqueForce=off  SenseLowerLimitTorqueForce=off  SenseUpperLimitTorqueForce=off  LowerLimitSpecify=on  LowerLimitBound=-0.802851455917  LowerLimitBoundUnits=rad  LowerLimitStiffness=1e4  LowerLimitStiffnessUnits=N*m/deg  LowerLimitDamping=10  LowerLimitDampingUnits=N*m/(deg/s)  LowerLimitTransitionRegionWidth=0.1  LowerLimitTransitionRegionWidthUnits=deg  UpperLimitSpecify=on  UpperLimitBound=0.802851455917  UpperLimitBoundUnits=rad  UpperLimitStiffness=1e4  UpperLimitStiffnessUnits=N*m/deg  UpperLimitDamping=10  UpperLimitDampingUnits=N*m/(deg/s)  UpperLimitTransitionRegionWidth=0.1  UpperLimitTransitionRegionWidthUnits=deg  PositionTargetSpecify=on  PositionTargetPriority=High  PositionTargetValue=0  PositionTargetValueUnits=rad  VelocityTargetSpecify=off  VelocityTargetPriority=Low  VelocityTargetValue=10  VelocityTargetValueUnits=deg/s
  FR_thigh : Subsystem
  FR_thigh_joint : sm_lib/Joints/Revolute Joint  JointMode=Normal  SenseConstraintForce=off  SenseConstraintForceX=off  SenseConstraintForceY=off  SenseConstraintForceZ=off  SenseConstraintTorque=off  SenseConstraintTorqueX=off  SenseConstraintTorqueY=off  SenseConstraintTorqueZ=off  SenseTotalForce=off  SenseTotalForceX=off  SenseTotalForceY=off  SenseTotalForceZ=off  SenseTotalTorque=off  SenseTotalTorqueX=off  SenseTotalTorqueY=off  SenseTotalTorqueZ=off  CompositeWrenchDir=FollowerOnBase  CompositeWrenchFrame=BaseFrame  EquilibriumPosition=0  EquilibriumPositionUnits=deg  SpringStiffness=0  SpringStiffnessUnits=N*m/deg  DampingCoefficient=0.01  DampingCoefficientUnits=kg*m^2/(rad*s)  TorqueActuationMode=ComputedTorque  MotionActuationMode=InputMotion  SensePosition=on  SenseVelocity=on  SenseAcceleration=on  SenseTorqueForce=off  SenseLowerLimitTorqueForce=off  SenseUpperLimitTorqueForce=off  LowerLimitSpecify=on  LowerLimitBound=-1.0471975512  LowerLimitBoundUnits=rad  LowerLimitStiffness=1e4  LowerLimitStiffnessUnits=N*m/deg  LowerLimitDamping=10  LowerLimitDampingUnits=N*m/(deg/s)  LowerLimitTransitionRegionWidth=0.1  LowerLimitTransitionRegionWidthUnits=deg  UpperLimitSpecify=on  UpperLimitBound=4.18879020479  UpperLimitBoundUnits=rad  UpperLimitStiffness=1e4  UpperLimitStiffnessUnits=N*m/deg  UpperLimitDamping=10  UpperLimitDampingUnits=N*m/(deg/s)  UpperLimitTransitionRegionWidth=0.1  UpperLimitTransitionRegionWidthUnits=deg  PositionTargetSpecify=on  PositionTargetPriority=High  PositionTargetValue=00.5938  PositionTargetValueUnits=rad  VelocityTargetSpecify=off  VelocityTargetPriority=High  VelocityTargetValue=1  VelocityTargetValueUnits=deg/s
  FR_thigh_shoulder : Subsystem
  PS-Simulink Converter{1..11} (11 alike) : nesl_utility/PS-Simulink Converter  PhysicalDomain=network_engine_domain  SubClassName=ps_output  LeftPortType=input  RightPortType=output  PseudoPeriodic=off  Frequencies=[]  VectorFormat=1-D array  Unit=inherit  AffineConversion=off
  Simulink-PS Converter : nesl_utility/Simulink-PS Converter  PhysicalDomain=network_engine_domain  SubClassName=ps_input  LeftPortType=input  RightPortType=output  PseudoPeriodic=off  Frequencies=[]  NoiseDistribution=none  NoiseParameters=[]  Unit=1  AffineConversion=off  FilteringAndDerivatives=filter  SimscapeFilterOrder=2  InputFilterTimeConstant=tc  UdotUserProvided=0
  Simulink-PS Converter1 : nesl_utility/Simulink-PS Converter  PhysicalDomain=network_engine_domain  SubClassName=ps_input  LeftPortType=input  RightPortType=output  PseudoPeriodic=off  Frequencies=[]  NoiseDistribution=none  NoiseParameters=[]  Unit=1  AffineConversion=off  FilteringAndDerivatives=filter  SimscapeFilterOrder=2  InputFilterTimeConstant=tc  UdotUserProvided=0
  Simulink-PS Converter2 : nesl_utility/Simulink-PS Converter  PhysicalDomain=network_engine_domain  SubClassName=ps_input  LeftPortType=input  RightPortType=output  PseudoPeriodic=off  Frequencies=[]  NoiseDistribution=none  NoiseParameters=[]  Unit=1  AffineConversion=off  FilteringAndDerivatives=filter  SimscapeFilterOrder=2  InputFilterTimeConstant=tc  UdotUserProvided=0
  Spatial Contact Force : sm_lib/Forces and Torques/Spatial Contact Force  SenseContactBaseRotation=off  SenseContactBaseTranslation=off  CoefficientOfDynamicFriction=1  CoefficientOfStaticFriction=1  NormalDamping=damp  NormalDampingUnits=N/(m/s)  SenseContactSignal=off  NormalStiffness=stiff  NormalStiffnessUnits=N/m  FrictionalCriticalVelocity=0.01  FrictionalCriticalVelocityUnits=m/s  ZeroCrossDetectContactStartAndEnd=off  SenseContactFollowerRotation=off  SenseContactFollowerTranslation=off  FrictionType=SmoothStickSlip  SenseFrictionalForceMagnitude=on  SenseNormalForceMagnitude=on  NormalForceType=SmoothSpringDamper  SenseNormalVelocity=off  SenseSeparationDistance=off  SenseTangentialVelocity=off  NormalTransitionRegionWidth=1e-4  NormalTransitionRegionWidthUnits=m
  C_FR : PMIOPort  Side=Left
  G_FR : PMIOPort  Port=2  Side=Left
  Fn_FR : Outport
  FFRM_FR : Outport  Port=2
  QS_HIP_FR : Outport  Port=3
  WS_HIP_FR : Outport  Port=4
  AS_HIP_FR : Outport  Port=5
  QS_THIGH_FR : Outport  Port=6
  WS_THIGH_FR : Outport  Port=7
  AS_THIGH_FR : Outport  Port=8
  QS_CALF_FR : Outport  Port=9
  WS_CALF_FR : Outport  Port=10
  AS_CALF_FR : Outport  Port=11
  wires:
  PS-Simulink Converter7/1 -> Fn_FR/1
  PS-Simulink Converter1/1 -> FFRM_FR/1
  PS-Simulink Converter2/1 -> QS_HIP_FR/1
  Q_HIP_FR/1 -> Simulink-PS Converter2/1
  PS-Simulink Converter3/1 -> WS_HIP_FR/1
  PS-Simulink Converter4/1 -> AS_HIP_FR/1
  PS-Simulink Converter5/1 -> QS_THIGH_FR/1
  PS-Simulink Converter8/1 -> AS_THIGH_FR/1
  PS-Simulink Converter6/1 -> WS_THIGH_FR/1
  PS-Simulink Converter11/1 -> QS_CALF_FR/1
  PS-Simulink Converter10/1 -> WS_CALF_FR/1
  PS-Simulink Converter9/1 -> AS_CALF_FR/1
  Q_CALF_FR/1 -> Simulink-PS Converter/1
  Q_THIGH_FR/1 -> Simulink-PS Converter1/1
  connections:
  FR_calf_joint/LConn1 -- FR_thigh/RConn1
  FR_calf/RConn1 -- FR_foot_fixed/LConn1
  FR_foot/LConn1 -- FR_foot_fixed/RConn1
  FR_thigh/LConn1 -- FR_thigh_joint/RConn1
  FR_hip_fixed/RConn1 -- FR_thigh_shoulder/LConn1
  FR_hip/RConn2 -- FR_hip_fixed/LConn1
  FR_calf/LConn1 -- FR_calf_joint/RConn1
  FR_hip/RConn1 -- FR_thigh_joint/LConn1
  FR_hip/LConn1 -- FR_hip_joint/RConn1
  FR_hip_joint/LConn1 -- C_FR/RConn1
  Spatial Contact Force/RConn2 -- PS-Simulink Converter7/LConn1
  PS-Simulink Converter1/LConn1 -- Spatial Contact Force/RConn3
  Spatial Contact Force/LConn1 -- G_FR/RConn1
  Spatial Contact Force/RConn1 -- FR_foot/LConn2
  FR_hip_joint/RConn2 -- PS-Simulink Converter2/LConn1
  Simulink-PS Converter2/RConn1 -- FR_hip_joint/LConn2
  FR_hip_joint/RConn3 -- PS-Simulink Converter3/LConn1
  FR_hip_joint/RConn4 -- PS-Simulink Converter4/LConn1
  FR_thigh_joint/RConn3 -- PS-Simulink Converter6/LConn1
  FR_thigh_joint/RConn4 -- PS-Simulink Converter8/LConn1
  Simulink-PS Converter1/RConn1 -- FR_thigh_joint/LConn2
  FR_thigh_joint/RConn2 -- PS-Simulink Converter5/LConn1
  FR_calf_joint/RConn2 -- PS-Simulink Converter11/LConn1
  Simulink-PS Converter/RConn1 -- FR_calf_joint/LConn2
  FR_calf_joint/RConn3 -- PS-Simulink Converter10/LConn1
  FR_calf_joint/RConn4 -- PS-Simulink Converter9/LConn1

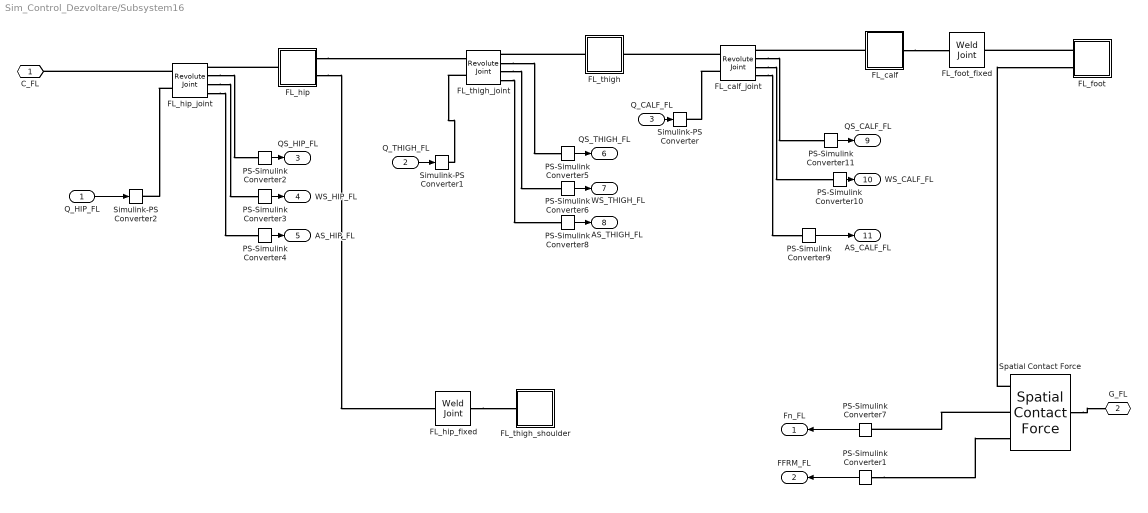
== system Sim_Control_Dezvoltare/Subsystem16 ==
  Q_HIP_FL : Inport
  Q_THIGH_FL : Inport  Port=2
  Q_CALF_FL : Inport  Port=3
  FL_calf : Subsystem
  FL_calf_joint : sm_lib/Joints/Revolute Joint  JointMode=Normal  SenseConstraintForce=off  SenseConstraintForceX=off  SenseConstraintForceY=off  SenseConstraintForceZ=off  SenseConstraintTorque=off  SenseConstraintTorqueX=off  SenseConstraintTorqueY=off  SenseConstraintTorqueZ=off  SenseTotalForce=off  SenseTotalForceX=off  SenseTotalForceY=off  SenseTotalForceZ=off  SenseTotalTorque=off  SenseTotalTorqueX=off  SenseTotalTorqueY=off  SenseTotalTorqueZ=off  CompositeWrenchDir=FollowerOnBase  CompositeWrenchFrame=BaseFrame  EquilibriumPosition=0  EquilibriumPositionUnits=deg  SpringStiffness=0  SpringStiffnessUnits=N*m/deg  DampingCoefficient=0.01  DampingCoefficientUnits=kg*m^2/(rad*s)  TorqueActuationMode=ComputedTorque  MotionActuationMode=InputMotion  SensePosition=on  SenseVelocity=on  SenseAcceleration=on  SenseTorqueForce=off  SenseLowerLimitTorqueForce=off  SenseUpperLimitTorqueForce=off  LowerLimitSpecify=on  LowerLimitBound=-2.69653369433  LowerLimitBoundUnits=rad  LowerLimitStiffness=1e4  LowerLimitStiffnessUnits=N*m/deg  LowerLimitDamping=10  LowerLimitDampingUnits=N*m/(deg/s)  LowerLimitTransitionRegionWidth=0.1  LowerLimitTransitionRegionWidthUnits=deg  UpperLimitSpecify=on  UpperLimitBound=-0.916297857297  UpperLimitBoundUnits=rad  UpperLimitStiffness=1e4  UpperLimitStiffnessUnits=N*m/deg  UpperLimitDamping=10  UpperLimitDampingUnits=N*m/(deg/s)  UpperLimitTransitionRegionWidth=0.1  UpperLimitTransitionRegionWidthUnits=deg  PositionTargetSpecify=on  PositionTargetPriority=High  PositionTargetValue=-1.7298  PositionTargetValueUnits=rad  VelocityTargetSpecify=off  VelocityTargetPriority=High  VelocityTargetValue=0  VelocityTargetValueUnits=deg/s
  FL_foot : Subsystem
  FL_foot_fixed : sm_lib/Joints/Weld Joint  JointMode=Normal  SenseConstraintForce=off  SenseConstraintForceX=off  SenseConstraintForceY=off  SenseConstraintForceZ=off  SenseConstraintTorque=off  SenseConstraintTorqueX=off  SenseConstraintTorqueY=off  SenseConstraintTorqueZ=off  SenseTotalForce=off  SenseTotalForceX=off  SenseTotalForceY=off  SenseTotalForceZ=off  SenseTotalTorque=off  SenseTotalTorqueX=off  SenseTotalTorqueY=off  SenseTotalTorqueZ=off  CompositeWrenchDir=FollowerOnBase  CompositeWrenchFrame=BaseFrame
  FL_hip : Subsystem
  FL_hip_fixed : sm_lib/Joints/Weld Joint  JointMode=Normal  SenseConstraintForce=off  SenseConstraintForceX=off  SenseConstraintForceY=off  SenseConstraintForceZ=off  SenseConstraintTorque=off  SenseConstraintTorqueX=off  SenseConstraintTorqueY=off  SenseConstraintTorqueZ=off  SenseTotalForce=off  SenseTotalForceX=off  SenseTotalForceY=off  SenseTotalForceZ=off  SenseTotalTorque=off  SenseTotalTorqueX=off  SenseTotalTorqueY=off  SenseTotalTorqueZ=off  CompositeWrenchDir=FollowerOnBase  CompositeWrenchFrame=BaseFrame
  FL_hip_joint : sm_lib/Joints/Revolute Joint  JointMode=Normal  SenseConstraintForce=off  SenseConstraintForceX=off  SenseConstraintForceY=off  SenseConstraintForceZ=off  SenseConstraintTorque=off  SenseConstraintTorqueX=off  SenseConstraintTorqueY=off  SenseConstraintTorqueZ=off  SenseTotalForce=off  SenseTotalForceX=off  SenseTotalForceY=off  SenseTotalForceZ=off  SenseTotalTorque=off  SenseTotalTorqueX=off  SenseTotalTorqueY=off  SenseTotalTorqueZ=off  CompositeWrenchDir=FollowerOnBase  CompositeWrenchFrame=BaseFrame  EquilibriumPosition=0  EquilibriumPositionUnits=deg  SpringStiffness=0  SpringStiffnessUnits=N*m/deg  DampingCoefficient=0.01  DampingCoefficientUnits=kg*m^2/(rad*s)  TorqueActuationMode=ComputedTorque  MotionActuationMode=InputMotion  SensePosition=on  SenseVelocity=on  SenseAcceleration=on  SenseTorqueForce=off  SenseLowerLimitTorqueForce=off  SenseUpperLimitTorqueForce=off  LowerLimitSpecify=on  LowerLimitBound=-0.802851455917  LowerLimitBoundUnits=rad  LowerLimitStiffness=1e4  LowerLimitStiffnessUnits=N*m/deg  LowerLimitDamping=10  LowerLimitDampingUnits=N*m/(deg/s)  LowerLimitTransitionRegionWidth=0.1  LowerLimitTransitionRegionWidthUnits=deg  UpperLimitSpecify=on  UpperLimitBound=0.802851455917  UpperLimitBoundUnits=rad  UpperLimitStiffness=1e4  UpperLimitStiffnessUnits=N*m/deg  UpperLimitDamping=10  UpperLimitDampingUnits=N*m/(deg/s)  UpperLimitTransitionRegionWidth=0.1  UpperLimitTransitionRegionWidthUnits=deg  PositionTargetSpecify=on  PositionTargetPriority=High  PositionTargetValue=0  PositionTargetValueUnits=rad  VelocityTargetSpecify=off  VelocityTargetPriority=High  VelocityTargetValue=0  VelocityTargetValueUnits=deg/s
  FL_thigh : Subsystem
  FL_thigh_joint : sm_lib/Joints/Revolute Joint  JointMode=Normal  SenseConstraintForce=off  SenseConstraintForceX=off  SenseConstraintForceY=off  SenseConstraintForceZ=off  SenseConstraintTorque=off  SenseConstraintTorqueX=off  SenseConstraintTorqueY=off  SenseConstraintTorqueZ=off  SenseTotalForce=off  SenseTotalForceX=off  SenseTotalForceY=off  SenseTotalForceZ=off  SenseTotalTorque=off  SenseTotalTorqueX=off  SenseTotalTorqueY=off  SenseTotalTorqueZ=off  CompositeWrenchDir=FollowerOnBase  CompositeWrenchFrame=BaseFrame  EquilibriumPosition=0  EquilibriumPositionUnits=deg  SpringStiffness=0  SpringStiffnessUnits=N*m/deg  DampingCoefficient=0.01  DampingCoefficientUnits=kg*m^2/(rad*s)  TorqueActuationMode=ComputedTorque  MotionActuationMode=InputMotion  SensePosition=on  SenseVelocity=on  SenseAcceleration=on  SenseTorqueForce=off  SenseLowerLimitTorqueForce=off  SenseUpperLimitTorqueForce=off  LowerLimitSpecify=on  LowerLimitBound=-1.0471975512  LowerLimitBoundUnits=rad  LowerLimitStiffness=1e4  LowerLimitStiffnessUnits=N*m/deg  LowerLimitDamping=10  LowerLimitDampingUnits=N*m/(deg/s)  LowerLimitTransitionRegionWidth=0.1  LowerLimitTransitionRegionWidthUnits=deg  UpperLimitSpecify=on  UpperLimitBound=4.18879020479  UpperLimitBoundUnits=rad  UpperLimitStiffness=1e4  UpperLimitStiffnessUnits=N*m/deg  UpperLimitDamping=10  UpperLimitDampingUnits=N*m/(deg/s)  UpperLimitTransitionRegionWidth=0.1  UpperLimitTransitionRegionWidthUnits=deg  PositionTargetSpecify=on  PositionTargetPriority=High  PositionTargetValue=0.5938  PositionTargetValueUnits=rad  VelocityTargetSpecify=off  VelocityTargetPriority=High  VelocityTargetValue=0  VelocityTargetValueUnits=deg/s
  FL_thigh_shoulder : Subsystem
  PS-Simulink Converter{1..11} (11 alike) : nesl_utility/PS-Simulink Converter  PhysicalDomain=network_engine_domain  SubClassName=ps_output  LeftPortType=input  RightPortType=output  PseudoPeriodic=off  Frequencies=[]  VectorFormat=1-D array  Unit=inherit  AffineConversion=off
  Simulink-PS Converter : nesl_utility/Simulink-PS Converter  PhysicalDomain=network_engine_domain  SubClassName=ps_input  LeftPortType=input  RightPortType=output  PseudoPeriodic=off  Frequencies=[]  NoiseDistribution=none  NoiseParameters=[]  Unit=1  AffineConversion=off  FilteringAndDerivatives=filter  SimscapeFilterOrder=2  InputFilterTimeConstant=tc  UdotUserProvided=0
  Simulink-PS Converter1 : nesl_utility/Simulink-PS Converter  PhysicalDomain=network_engine_domain  SubClassName=ps_input  LeftPortType=input  RightPortType=output  PseudoPeriodic=off  Frequencies=[]  NoiseDistribution=none  NoiseParameters=[]  Unit=1  AffineConversion=off  FilteringAndDerivatives=filter  SimscapeFilterOrder=2  InputFilterTimeConstant=tc  UdotUserProvided=0
  Simulink-PS Converter2 : nesl_utility/Simulink-PS Converter  PhysicalDomain=network_engine_domain  SubClassName=ps_input  LeftPortType=input  RightPortType=output  PseudoPeriodic=off  Frequencies=[]  NoiseDistribution=none  NoiseParameters=[]  Unit=1  AffineConversion=off  FilteringAndDerivatives=filter  SimscapeFilterOrder=2  InputFilterTimeConstant=tc  UdotUserProvided=0
  Spatial Contact Force : sm_lib/Forces and Torques/Spatial Contact Force  SenseContactBaseRotation=off  SenseContactBaseTranslation=off  CoefficientOfDynamicFriction=1  CoefficientOfStaticFriction=1  NormalDamping=damp  NormalDampingUnits=N/(m/s)  SenseContactSignal=off  NormalStiffness=stiff  NormalStiffnessUnits=N/m  FrictionalCriticalVelocity=0.01  FrictionalCriticalVelocityUnits=m/s  ZeroCrossDetectContactStartAndEnd=off  SenseContactFollowerRotation=off  SenseContactFollowerTranslation=off  FrictionType=SmoothStickSlip  SenseFrictionalForceMagnitude=on  SenseNormalForceMagnitude=on  NormalForceType=SmoothSpringDamper  SenseNormalVelocity=off  SenseSeparationDistance=off  SenseTangentialVelocity=off  NormalTransitionRegionWidth=1e-4  NormalTransitionRegionWidthUnits=m
  C_FL : PMIOPort  Side=Left
  G_FL : PMIOPort  Port=2  Side=Left
  Fn_FL : Outport
  FFRM_FL : Outport  Port=2
  QS_HIP_FL : Outport  Port=3
  WS_HIP_FL : Outport  Port=4
  AS_HIP_FL : Outport  Port=5
  QS_THIGH_FL : Outport  Port=6
  WS_THIGH_FL : Outport  Port=7
  AS_THIGH_FL : Outport  Port=8
  QS_CALF_FL : Outport  Port=9
  WS_CALF_FL : Outport  Port=10
  AS_CALF_FL : Outport  Port=11
  wires:
  PS-Simulink Converter7/1 -> Fn_FL/1
  PS-Simulink Converter1/1 -> FFRM_FL/1
  PS-Simulink Converter2/1 -> QS_HIP_FL/1
  PS-Simulink Converter3/1 -> WS_HIP_FL/1
  PS-Simulink Converter4/1 -> AS_HIP_FL/1
  Q_HIP_FL/1 -> Simulink-PS Converter2/1
  PS-Simulink Converter5/1 -> QS_THIGH_FL/1
  PS-Simulink Converter8/1 -> AS_THIGH_FL/1
  PS-Simulink Converter6/1 -> WS_THIGH_FL/1
  Q_THIGH_FL/1 -> Simulink-PS Converter1/1
  Q_CALF_FL/1 -> Simulink-PS Converter/1
  PS-Simulink Converter9/1 -> AS_CALF_FL/1
  PS-Simulink Converter10/1 -> WS_CALF_FL/1
  PS-Simulink Converter11/1 -> QS_CALF_FL/1
  connections:
  FL_calf_joint/LConn1 -- FL_thigh/RConn1
  FL_foot/LConn1 -- FL_foot_fixed/RConn1
  FL_calf/RConn1 -- FL_foot_fixed/LConn1
  FL_thigh/LConn1 -- FL_thigh_joint/RConn1
  FL_calf/LConn1 -- FL_calf_joint/RConn1
  FL_hip/LConn1 -- FL_hip_joint/RConn1
  FL_hip/RConn1 -- FL_thigh_joint/LConn1
  FL_hip/RConn2 -- FL_hip_fixed/LConn1
  FL_hip_fixed/RConn1 -- FL_thigh_shoulder/LConn1
  FL_hip_joint/LConn1 -- C_FL/RConn1
  Spatial Contact Force/RConn2 -- PS-Simulink Converter7/LConn1
  PS-Simulink Converter1/LConn1 -- Spatial Contact Force/RConn3
  Spatial Contact Force/LConn1 -- G_FL/RConn1
  Spatial Contact Force/RConn1 -- FL_foot/LConn2
  FL_hip_joint/RConn3 -- PS-Simulink Converter3/LConn1
  FL_hip_joint/RConn4 -- PS-Simulink Converter4/LConn1
  FL_hip_joint/RConn2 -- PS-Simulink Converter2/LConn1
  FL_hip_joint/LConn2 -- Simulink-PS Converter2/RConn1
  FL_thigh_joint/RConn2 -- PS-Simulink Converter5/LConn1
  FL_thigh_joint/LConn2 -- Simulink-PS Converter1/RConn1
  FL_thigh_joint/RConn3 -- PS-Simulink Converter6/LConn1
  FL_thigh_joint/RConn4 -- PS-Simulink Converter8/LConn1
  FL_calf_joint/RConn2 -- PS-Simulink Converter11/LConn1
  FL_calf_joint/RConn4 -- PS-Simulink Converter9/LConn1
  FL_calf_joint/RConn3 -- PS-Simulink Converter10/LConn1
  FL_calf_joint/LConn2 -- Simulink-PS Converter/RConn1

== system Sim_Control_Dezvoltare/Subsystem17 ==
  MechanismConfiguration : sm_lib/Utilities/Mechanism Configuration  UniformGravity=Constant  GravityVector=[0 0 -9.80665]  GravityUnits=m/s^2  LinearizationDelta=0.001  JointModeTransitionNonlinearIterations=2
  Solver Configuration : nesl_utility/Solver Configuration  PhysicalDomain=network_engine_domain  SubClassName=solver  LeftPortType=input  RightPortType=generic  Tones=[]  Harmonics=[]  SimulateNoise=off  Profile=off  UseLocalSampling=off  EnableSwitchedLinearOptims=on  FrequencyDomain=off  UseCCode=off  RelTol=0.001  AbsTol=0.001  MinStep=1e-09  ToWorkspace=off  RevertToSquareIcSolve=off  NumHomotopyIterations=100  PhasorMode=off  PhasorModeNumHarmonics=1  ConsistencySolver=NEWTON_FTOL  IndexReductionMethod=DerivativeReplacement  DoDC=off  ResidualTolerance=1e-09  ConsistencyTolSource=GLOBAL  ConsistencyAbsTol=0.001  ConsistencyRelTol=0.001  ConsistencyTolFactor=0.001  UseLocalSolver=off  LocalSolverChoice=NE_BACKWARD_EULER_ADVANCER  ResolveIndetEquations=on  FunctionEvalNumThread=1  LocalSolverSampleTime=0.001  DoFixedCost=off  MaxNonlinIter=3  MaxModeIter=2  ComputeImpulses=off  ImpulseIterations=2  LinearAlgebra=auto  LinearAlgebraNumThread=0  EquationFormulation=NE_TIME_EF  DelaysMemoryBudget=1024  AutomaticFiltering=on  FilteringTimeConstant=0.001  PartitionStorageMethod=AS_NEEDED  PartitionMemoryBudget=1024  PartitionMethod=ROBUST
  Trajectory Display : sm_lib/Curves and Surfaces/Spline  GraphicAmbientColor=[0.15 0.15 0.15 1.0]  GraphicDiffuseColor=[0 0 0]  DataPoints=interPts  DataPointsUnits=m  GraphicEmissiveColor=[0.0 0.0 0.0 1.0]  EndConditionType=Natural  MarkerShape=Sphere  MarkerSize=10  GraphicType=FromGeometry  GraphicOpacity=1.0  GraphicShininess=75  GraphicSpecularColor=[0.5 0.5 0.5 1.0]  GraphicVisPropType=SimpleVisualProperties
  Transform Floor Frame : sm_lib/Frames and Transforms/Rigid Transform  TranslationMethod=StandardAxis  TranslationStandardOffset=-0.06  TranslationLengthUnit=m  TranslationStandardAxis=+Z  TranslationCartesianOffset=[0 0 0]  TranslationROffset=0  TranslationROffsetUnits=m  TranslationZOffset=0  TranslationZOffsetUnits=m  TranslationThetaOffset=0  TranslationThetaOffsetUnits=deg  RotationMethod=None  RotationAngleUnits=deg  RotationStandardAxis=+X  RotationAngle=-90  RotationArbitraryAxis=[0 0 1]  FollAlignAxisA=+X  BaseAlignAxisA=+Y  FollAlignAxisB=+Y  BaseAlignAxisB=+Z  RotationSequenceAxes=FollowerAxes  RotationSequence=XYX  RotationSequenceAngles=[0 0 0]  RotationSequenceAnglesUnits=deg  RotationMatrix=[1 0 0; 0 1 0; 0 0 1]  Quaternion=[1 0 0 0]
  World : sm_lib/Frames and Transforms/World Frame
  World Plane : sm_lib/Body Elements/Brick Solid  GraphicAmbientColor=[0.15 0.15 0.15 1.0]  BasedOnType=Density  BrickDimensions=[15 15 0.1]  BrickDimensionUnits=m  CenterOfMass=[0 0 0]  CenterOfMassUnits=m  GraphicDiffuseColor=[0.2 0.2 1.0]  Density=1000  DensityUnits=kg/(m^3)  DoExposeReferenceFrame=on  GraphicEmissiveColor=[0.0 0.0 0.0 1.0]  ExportEntireGeometry=on  SerializedFrames=<Frames/>  MarkerShape=Sphere  MarkerSize=10  GraphicType=FromGeometry  InertiaType=CalculateFromGeometry  Mass=1  MassUnits=kg  MomentsOfInertia=[1 1 1]  MomentsOfInertiaUnits=kg*m^2  GraphicOpacity=0.5  ProductsOfInertia=[0 0 0]  ProductsOfInertiaUnits=kg*m^2  GraphicShininess=75  GraphicSpecularColor=[0.5 0.5 0.5 1.0]  GraphicVisPropType=SimpleVisualProperties
  G : PMIOPort  Side=Left
  W : PMIOPort  Port=2  Side=Left
  connections:
  Transform Floor Frame/LConn1 -- Solver Configuration/RConn1 -- MechanismConfiguration/RConn1 -- Trajectory Display/LConn1 -- W/RConn1 -- World/RConn1
  World Plane/RConn1 -- Transform Floor Frame/RConn1
  World Plane/LConn1 -- G/RConn1
